simulink model "CanSat_BaseStation_Model3"  (R2022b)
settings: Solver=VariableStepAuto  StartTime=0.0  StopTime=20  RelTol=1e-3
undefined symbols (not defined in the file): fdesignblkfcn, gcbh
libraries: dspsnks4 x1, dspmlti4 x1, sdrrlib x1
settings Model: Creator=caryc  LastModifiedBy=caryc

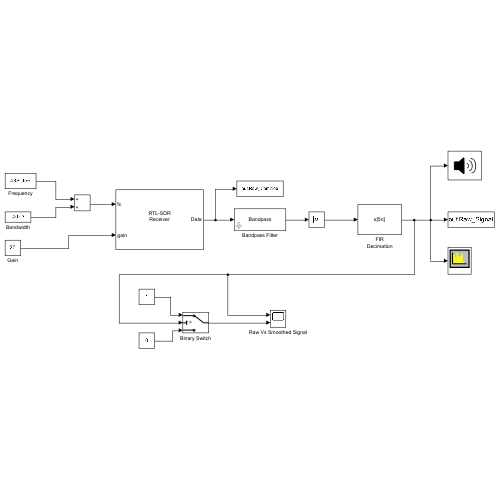
[thumbnail: Simulink's stored preview of the top-level diagram]
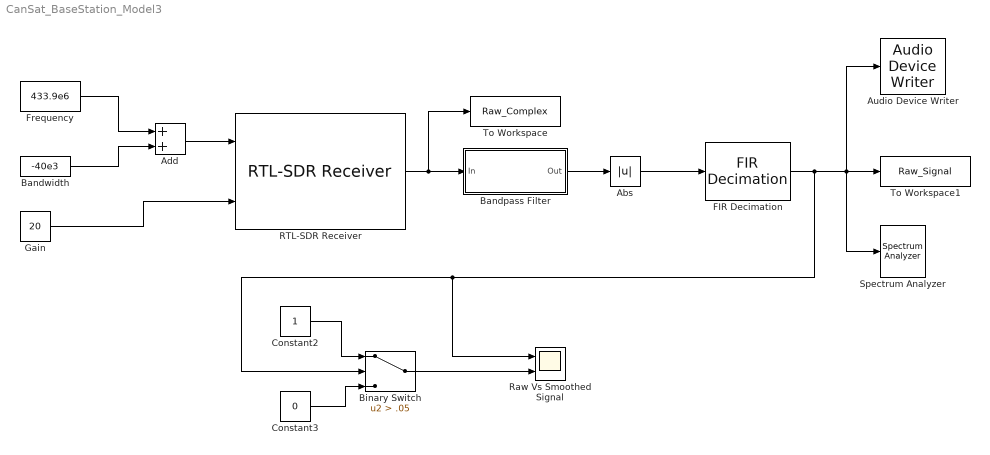
== system CanSat_BaseStation_Model3 ==
  Abs : Abs  SaturateOnIntegerOverflow=off
  Add : Sum
  Audio Device Writer : dspsnks4/Audio Device Writer  Driver=DirectSound  Device=Default  InheritSampleRate=on  SampleRate=44100  BitDepth=16-bit integer  BufferSize=4096  NumBuffers=10  DefaultOutputChannelMapping=on  OutputChannelMapping=1:2  OutputNumUnderrunSamples=off  DriverIdx=1  DeviceWarnFlag=''
  Bandpass Filter : Subsystem  DialogController=fdesignblkfcn  InitFcn=fdesignblkfcn(gcbh, {'InitFcn'});  mask(Bandpass Filter){}
      mask help: Design a bandpass filter
      settings: CopyFcn=fdesignblkfcn(gcbh, {'CopyFcn'});
      mask Help: helpview(mapfilelocation('dsp'), 'dspbandpassfilter');
      mask Display: disp('Bandpass');
  Bandwidth : Constant  Value=-40e3
  Binary Switch : Switch  Criteria=u2 > Threshold  Threshold=.05  SaturateOnIntegerOverflow=off
  Constant2 : Constant
  Constant3 : Constant  Value=0
  FIR Decimation : dspmlti4/FIR Decimation  FilterSource=Dialog parameters  h=firpm(100, [0 15e3 20e3 (240e3/2)]/(240e3/2), [1 1 0 0], [1 1], 20)  D=5  filtStruct=Direct form  FilterObject=FDECIM  InputProcessing=Columns as channels (frame based)  framing=Allow multirate processing  AllowArbitraryInputLength=off  inputOffset=0  outputBufInitCond=0  roundingMode=Floor  overflowMode=off  firstCoeffDataTypeStr=Inherit: Same word length as input  firstCoeffMin=[]  firstCoeffMax=[]  firstCoeffLastDataTypeStr=Inherit: Same word length as input  outputDataTypeStr=Inherit: Same as accumulator  outputMin=[]  outputMax=[]  outputLastDataTypeStr=Inherit: Same as accumulator
      settings: LibrarySourceBlock=|
      | dsphdlsupportfiltering/FIR
      | Decimation
  Frequency : Constant  Value=433.9e6
  Gain : Constant  Value=20
  RTL-SDR Receiver : sdrrlib/RTL-SDR Receiver  IPAddress=0  CenterFrequencySource=Input port  CenterFrequency=102.5e6  GainSource=Input port  Gain=0  ADCRate=250e3  FrequencyCorrection=0  LostSamplesOutputPort=off  LatencyOutputPort=off  OutputDataType=double  FrameLength=1024  EnableBurstMode=off  NumFramesInBurst=20  sobjType=sdrr.internal.SDRRTLReceiverSL  dataUDPPort=-1  ctrlUDPPort=-1  subDeviceList=nosubdev  sdrBlockType=SDRBlockTypeSLT.SDRRxBlock  requester=UNUSED_BY_SFCN  sdrExecutionMode=SDRExecutionModeSLT.ExecModeHW  BypassUserLogic=off  DecimatorSelect=DDC decimator  SourceSelect=RF data  SineAmplitude=16000  EnableInternalClock=off  BypassIQBalance=off  IFBandwidth=40e6  ADCRateSource=Dialog  IntermediateFrequency=0  DecimationFactorSource=Dialog  DecimationFactor=512  RFFrequencyIsTunable=logical(1)  SampleTime=(1024)/(250e3)  IFBandwidthSource=Dialog  SineFrequency=30000  BypassDCBlockingFilter=off  IntermediateFrequencySource=Dialog  IQBalanceCoefficients=64  SkipAllHardwareResetAndInitialization=off  EnableIQCalibrationTable=on  CacheIQCalibrationTable=off  EnableOffsetTuning=off  EnableRTLAGC=off  EnableTestMode=off  EnableTunerAGC=off  FrequencyCorrectionSource=Dialog  NumMLBuffers=128  NumUSBBuffers=16  RTLCrystalFrequency=28800000  TunerCrystalFrequency=28800000
  Raw Vs Smoothed Signal : Scope  NumInputPorts=2
  Spectrum Analyzer : SpectrumAnalyzer
  To Workspace : ToWorkspace  VariableName=Raw_Complex  SampleTime=-1
      settings: Save2DSignal=2-D array (concatenate along first dimension)
  To Workspace1 : ToWorkspace  VariableName=Raw_Signal  SaveFormat=Timeseries  SampleTime=-1
  wires:
  Add/1 -> RTL-SDR Receiver/1
  Frequency/1 -> Add/1
  Bandwidth/1 -> Add/2
  Gain/1 -> RTL-SDR Receiver/2
  RTL-SDR Receiver/1 -> To Workspace/1, Bandpass Filter/1(In)
  Bandpass Filter/1(Out) -> Abs/1
  Abs/1 -> FIR Decimation/1
  Constant3/1 -> Binary Switch/3
  Constant2/1 -> Binary Switch/1
  Binary Switch/1 -> Raw Vs Smoothed Signal/2
  FIR Decimation/1 -> To Workspace1/1, Audio Device Writer/1, Spectrum Analyzer/1, Raw Vs Smoothed Signal/1, Binary Switch/2

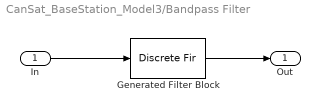
== system CanSat_BaseStation_Model3/Bandpass Filter ==
  In : Inport
  Generated Filter Block : DiscreteFir  Tag=BlockMethodSubSystem  Coefficients=[0.0024383680654391322 -0.00249048448723352116 0.000829618158799000707 0.000757639909411926137 -0.00297439999954760264 -0.00569567554311764448 -0.00287769587371433525 0.00202335772559120251 0.00233106594051531689 -0.000272122046722714206 0.0012989807907630524 0.00555508782838593472 0.00373686660212212965 -0.00370775607690403434 -0.00613059502047849127 -0.00156733498646653029 -0.00064541981755782032 -0.00588533303396905367 -0.00497548071923391722 0.00605849467576977715 0.0121345681081407326 0.00468287519693485858 -0.0019634302976165724 0.00305830740492445087 0.00523359569682744444 -0.00815203734622665238 -0.0196345055166754281 -0.00950525822702420579 0.00684044207879411486 0.00478878751753836381 -0.00332884812683291323 0.00909523350079553469 0.0276394504169403844 0.0161920213367104382 -0.0150761219722256763 -0.0210983733622466738 -0.0027404495183461562 -0.00715859816730031809 -0.0348113060828855736 -0.0258326425539628264 0.0299326964811326354 0.0565084056002555166 0.019341104119483532 -0.00294076064128450439 0.0397881049420063942 0.0472987256841347486 -0.0761641288587477649 -0.207207484433210409 -0.1261020839049386 0.14072053470827206 0.291759208615674559 0.14072053470827206 -0.1261020839049386 -0.207207484433210409 -0.0761641288587477649 0.0472987256841347486 0.0397881049420063942 -0.00294076064128450439 0.019341104119483532 0.0565084056002555166 0.0299326964811326354 -0.0258326425539628264 -0.0348113060828855736 -0.00715859816730031809 -0.0027404495183461562 -0.0210983733622466738 -0.0150761219722256763 0.0161920213367104382 0.0276394504169403844 0.00909523350079553469 -0.00332884812683291323 0.00478878751753836381 0.00684044207879411486 -0.00950525822702420579 -0.0196345055166754281 -0.00815203734622665238 0.00523359569682744444 0.00305830740492445087 -0.0019634302976165724 0.00468287519693485858 0.0121345681081407326 0.00605849467576977715 -0.00497548071923391722 -0.00588533303396905367 -0.00064541981755782032 -0.00156733498646653029 -0.00613059502047849127 -0.00370775607690403434 0.00373686660212212965 0.00555508782838593472 0.0012989807907630524 -0.000272122046722714206 0.00233106594051531689 0.00202335772559120251 -0.00287769587371433525 -0.00569567554311764448 -0.00297439999954760264 0.000757639909411926137 0.000829618158799000707 -0.00249048448723352116 0.0024383680654391322]  InputProcessing=Columns as channels (frame based)
  Out : Outport  VectorParamsAs1DForOutWhenUnconnected=off
  wires:
  In/1 -> Generated Filter Block/1
  Generated Filter Block/1 -> Out/1
